simulink model "calk"  (R2022a)
settings: Solver=VariableStepAuto  StartTime=0.0  StopTime=10.0  RelTol=1e-3
settings Model: Creator=Vova  LastModifiedBy=Vova

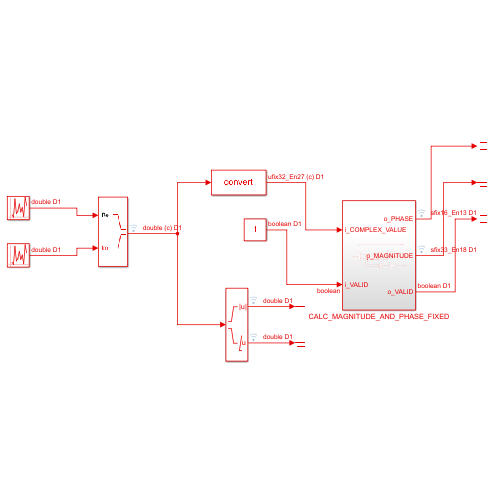
[thumbnail: Simulink's stored preview of the top-level diagram]
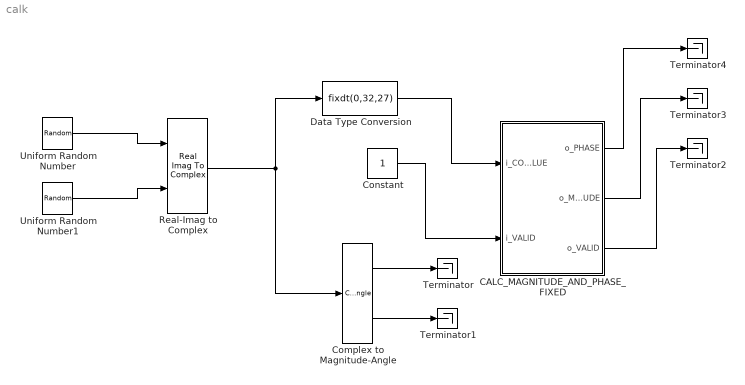
== system calk ==
  CALC_MAGNITUDE_AND_PHASE_FIXED : Subsystem
  Complex to Magnitude-Angle : ComplexToMagnitudeAngle
  Constant : Constant  OutDataTypeStr=boolean  SampleTime=1
  Data Type Conversion : DataTypeConversion  OutDataTypeStr=fixdt(0,32,27)  RndMeth=Round  SaturateOnIntegerOverflow=off
  Real-Imag to Complex : RealImagToComplex
  Terminator{,1..4} (5 alike) : Terminator
  Uniform Random Number : UniformRandomNumber  Minimum=0  Maximum=31.9999999254941940308  Seed=5  SampleTime=1
  Uniform Random Number1 : UniformRandomNumber  Minimum=0  Maximum=31.9999999254941940308  Seed=6  SampleTime=1
  wires:
  Real-Imag to Complex/1 -> Data Type Conversion/1, Complex to Magnitude-Angle/1
  Complex to Magnitude-Angle/1 -> Terminator/1
  CALC_MAGNITUDE_AND_PHASE_FIXED/2(o_MAGNITUDE) -> Terminator3/1
  Complex to Magnitude-Angle/2 -> Terminator1/1
  Uniform Random Number/1 -> Real-Imag to Complex/1
  Constant/1 -> CALC_MAGNITUDE_AND_PHASE_FIXED/2(i_VALID)
  CALC_MAGNITUDE_AND_PHASE_FIXED/3(o_VALID) -> Terminator2/1
  Data Type Conversion/1 -> CALC_MAGNITUDE_AND_PHASE_FIXED/1(i_COMPLEX_VALUE)
  Uniform Random Number1/1 -> Real-Imag to Complex/2
  CALC_MAGNITUDE_AND_PHASE_FIXED/1(o_PHASE) -> Terminator4/1

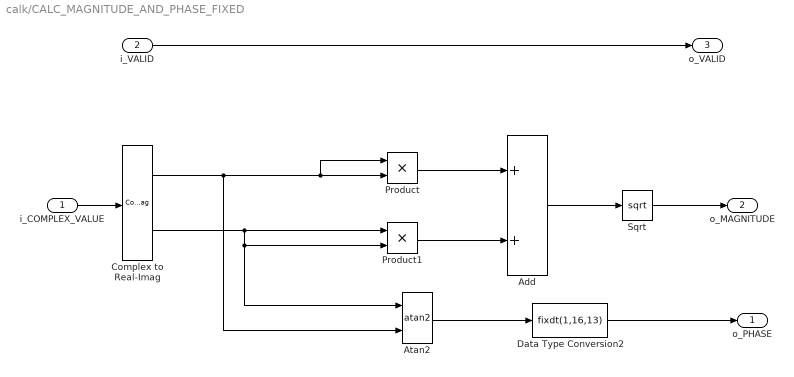
== system calk/CALC_MAGNITUDE_AND_PHASE_FIXED ==
  i_COMPLEX_VALUE : Inport
  i_VALID : Inport  Port=2  OutDataTypeStr=boolean
  Add : Sum  OutDataTypeStr=fixdt(0,65,55)
  Atan2 : Trigonometry  Operator=atan2  ApproximationMethod=CORDIC  NumberOfIterations=30
  Complex to Real-Imag : ComplexToRealImag
  Data Type Conversion2 : DataTypeConversion  OutDataTypeStr=fixdt(1,16,13)  SaturateOnIntegerOverflow=off  RndMeth=Floor
  Product : Product  OutDataTypeStr=fixdt(1, 64, 54)  SaturateOnIntegerOverflow=on
  Product1 : Product  OutDataTypeStr=fixdt(1, 64, 54)  LockScale=on
  Sqrt : Sqrt  OutDataTypeStr=fixdt(1,33,18)
  o_PHASE : Outport
  o_MAGNITUDE : Outport  Port=2
  o_VALID : Outport  Port=3  OutDataTypeStr=boolean
  wires:
  Complex to Real-Imag/2 -> Product1/1, Atan2/1, Product1/2
  Complex to Real-Imag/1 -> Atan2/2, Product/1, Product/2
  Atan2/1 -> Data Type Conversion2/1
  Data Type Conversion2/1 -> o_PHASE/1
  Product1/1 -> Add/2
  Product/1 -> Add/1
  Add/1 -> Sqrt/1
  Sqrt/1 -> o_MAGNITUDE/1
  i_COMPLEX_VALUE/1 -> Complex to Real-Imag/1
  i_VALID/1 -> o_VALID/1
